simulink model "power_Transformations"  (R2021a)
settings: Solver=ode45  StartTime=0.0  StopTime=0.05  MaxStep=50e-6  RelTol=1e-3  EnableMultiTasking=on
PreLoadFcn:
  | Ts=50e-6;
InitFcn:
  | if ~exist('Ts','var')
  | Ts=50e-6;
  | end
libraries: spsAlphaBetaZerotoabcLib x2, spsAlphaBetaZerotodq0Lib x2, spsabctoAlphaBetaZeroLib x2, spsdq0toAlphaBetaZeroLib x2, spsThreePhaseProgrammableGeneratorLib x1, spsabctodq0Lib x1, spsdq0toabcLib x1, simulink x1
settings Model: Creator=The MathWorks, Inc.  LastModifiedBy=User
settings SolverCC: AlgebraicLoopSolver=TrustRegion
settings DataIOCC: LimitDataPoints=on  SaveFormat=Array  SaveOutput=off  SaveTime=off  ReturnWorkspaceOutputs=off
settings OptimizationCC: ExpressionDepthLimit=2147483647  LifeSpan=inf
settings DebuggingCC: UnderspecifiedInitializationDetection=Classic  MergeDetectMultiDrivingBlocksExec=none  FcnCallInpInsideContextMsg=warning  StateNameClashWarn=warning  SFUnexpectedBacktrackingDiag=warning  SFNoUnconditionalDefaultTransitionDiag=warning  SFExecutionAtInitializationDiag=none  SFMachineParentedDataDiag=warning  ArithmeticOperatorsInVariantConditions=warning
settings HardwareCC: ProdBitPerPointer=32  ProdBitPerSizeT=32  ProdBitPerPtrDiffT=32  ProdLargestAtomicFloat=None  ProdIntDivRoundTo=Undefined  ProdEndianess=Unspecified  ProdWordSize=32  ProdHWDeviceType=32-bit Generic
settings ModelReferenceCC: PropagateSignalLabelsOutOfModel=off
settings SFSimCC: SimUseLocalCustomCode=off  CustomCodeUndefinedFunction=UseInterfaceOnly
settings RTWCC: RTWUseLocalCustomCode=off
settings CodeAppCC: StateflowObjectComments=on
settings GRTTargetCC: TargetLangStandard=C89/C90 (ANSI)  CombineOutputUpdateFcns=off  GRTInterface=on
settings ConfigComp: CovMetricSettings=dw  CovSaveCumulativeToWorkspaceVar=on  CovSaveSingleToWorkspaceVar=on  CovExternalEMLEnable=off  CovSFcnEnable=off

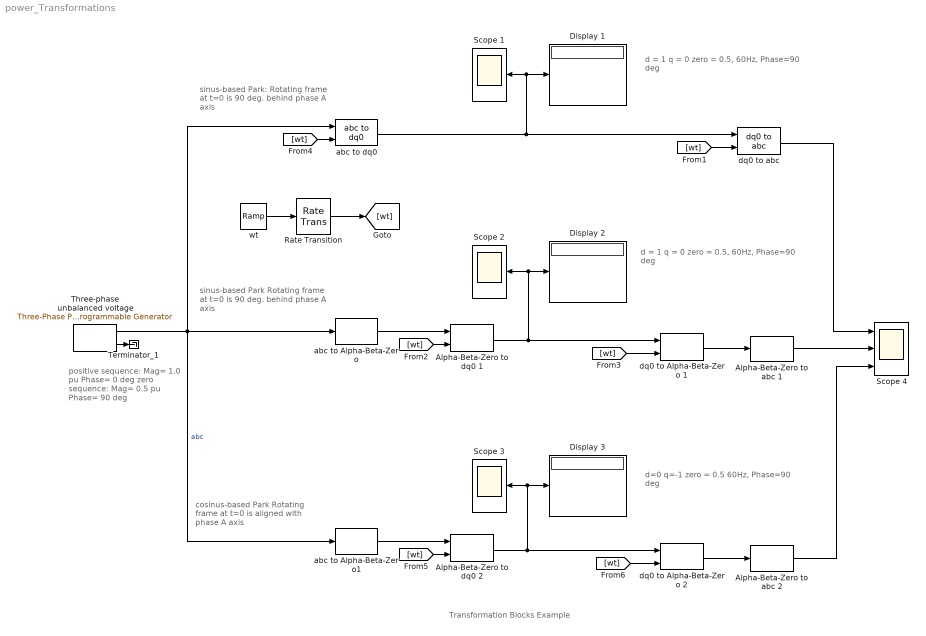
== system power_Transformations ==
  note: positive sequence:
      |    Mag= 1.0 pu
      |    Phase= 0 deg
      |
      | zero sequence:
      |    Mag= 0.5 pu
      |    Phase= 90 deg
  note: d = 1
      | q = 0
      | zero = 0.5,  60Hz,  Phase=90 deg
  note: cosinus-based Park
      | Rotating frame at t=0 is
      | aligned with phase A axis
  note: d=0
      | q=-1
      | zero = 0.5  60Hz,  Phase=90 deg
  note: sinus-based Park:
      | Rotating frame at t=0 is
      | 90 deg. behind phase A axis
  note: d = 1
      | q = 0
      | zero = 0.5,  60Hz,  Phase=90 deg
  note: sinus-based Park
      | Rotating frame at t=0 is
      | 90 deg. behind phase A axis
  note: Transformation Blocks Example
  Alpha-Beta-Zero to abc 1 : spsAlphaBetaZerotoabcLib/Alpha-Beta-Zero to abc
      settings: SourceProductBaseCode=PS
  Alpha-Beta-Zero to abc 2 : spsAlphaBetaZerotoabcLib/Alpha-Beta-Zero to abc
      settings: SourceProductBaseCode=PS
  Alpha-Beta-Zero to dq0 1 : spsAlphaBetaZerotodq0Lib/Alpha-Beta-Zero to dq0  Alignment=90 degrees behind phase A axis
      settings: SourceProductBaseCode=PS
  Alpha-Beta-Zero to dq0 2 : spsAlphaBetaZerotodq0Lib/Alpha-Beta-Zero to dq0  Alignment=Aligned with phase A axis
      settings: SourceProductBaseCode=PS
  Display 1 : Display
      settings: Format=bank
  Display 2 : Display
      settings: Format=bank
  Display 3 : Display
      settings: Format=bank
  Rate Transition : RateTransition  OutPortSampleTime=Ts
  Scope 1 : Scope
  Scope 2 : Scope
  Scope 3 : Scope
  Scope 4 : Scope  NumInputPorts=3
  Terminator_1 : Terminator
  Three-phase unbalanced voltage : spsThreePhaseProgrammableGeneratorLib/Three-Phase Programmable Generator  Par_Vps="[1  0 60]"  VariationEntity=None  VariationType=Ramp  VariationStep=-0.5  VariationRate=10  VariationMag=0.3  VariationFreq=2  Par_Timing_Variation="[0.2  1.2]"  SinglePhase=on  Yampli=[1 0.2 1.2 1.0]  Xtime=[0 0.1 0.15 0.2]  HarmonicGeneration=on  Par_HarmoA="[1  0.5  90  0]"  Par_HarmoB="[1  0  0   2]"  Par_Timing_Harmo="[ 0  99]"  Ts=Ts
      settings: SourceProductBaseCode=PS
  abc to Alpha-Beta-Zero : spsabctoAlphaBetaZeroLib/abc to Alpha-Beta-Zero
      settings: SourceProductBaseCode=PS
  abc to Alpha-Beta-Zero1 : spsabctoAlphaBetaZeroLib/abc to Alpha-Beta-Zero
      settings: SourceProductBaseCode=PS
  abc to dq0 : spsabctodq0Lib/abc to dq0  Alignment=90 degrees behind phase A axis
  dq0 to Alpha-Beta-Zero 1 : spsdq0toAlphaBetaZeroLib/dq0 to Alpha-Beta-Zero  Alignment=90 degrees behind phase A axis
      settings: SourceProductBaseCode=PS
  dq0 to Alpha-Beta-Zero 2 : spsdq0toAlphaBetaZeroLib/dq0 to Alpha-Beta-Zero  Alignment=Aligned with phase A axis
      settings: SourceProductBaseCode=PS
  dq0 to abc : spsdq0toabcLib/dq0 to abc  Alignment=90 degrees behind phase A axis
  wt : simulink/Sources/Ramp  slope=2*pi*60  start=0  InitialOutput=0
  wires:
  wt/1 -> Rate Transition/1
  abc to Alpha-Beta-Zero/1 -> Alpha-Beta-Zero to dq0 1/1
  abc to dq0/1 -> Scope 1/1, Display 1/1, dq0 to abc/1
  Alpha-Beta-Zero to dq0 1/1 -> dq0 to Alpha-Beta-Zero 1/1, Display 2/1, Scope 2/1
  dq0 to Alpha-Beta-Zero 1/1 -> Alpha-Beta-Zero to abc 1/1
  Alpha-Beta-Zero to dq0 2/1 -> Display 3/1, Scope 3/1, dq0 to Alpha-Beta-Zero 2/1
  dq0 to Alpha-Beta-Zero 2/1 -> Alpha-Beta-Zero to abc 2/1
  Rate Transition/1 -> [wt]
  [wt] -> abc to dq0/2
  [wt] -> dq0 to abc/2
  abc to Alpha-Beta-Zero1/1 -> Alpha-Beta-Zero to dq0 2/1
  [wt] -> Alpha-Beta-Zero to dq0 1/2
  [wt] -> dq0 to Alpha-Beta-Zero 1/2
  [wt] -> Alpha-Beta-Zero to dq0 2/2
  [wt] -> dq0 to Alpha-Beta-Zero 2/2
  Three-phase unbalanced voltage/1 -> abc to Alpha-Beta-Zero1/1, abc to dq0/1, abc to Alpha-Beta-Zero/1  "abc"
  dq0 to abc/1 -> Scope 4/1
  Alpha-Beta-Zero to abc 1/1 -> Scope 4/2
  Alpha-Beta-Zero to abc 2/1 -> Scope 4/3
  Three-phase unbalanced voltage/2 -> Terminator_1/1
